simulink model "TP7"  (R2023b)
settings: Solver=VariableStepAuto  StartTime=0.0  StopTime=0.4  RelTol=1e-3
libraries: spsMosfetLib x6, spsSeriesRLCBranchLib x3, spsVoltageMeasurementLib x3, spsGroundLib x2, spsDCVoltageSourceLib x1, dspstat3 x1, sps_lib x1
settings Model: Creator=HP  LastModifiedBy=HP

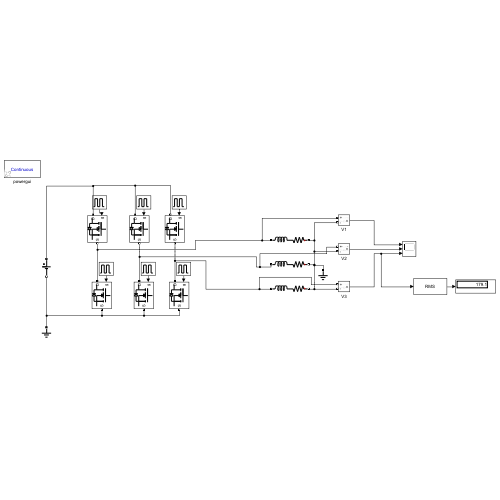
[thumbnail: Simulink's stored preview of the top-level diagram]
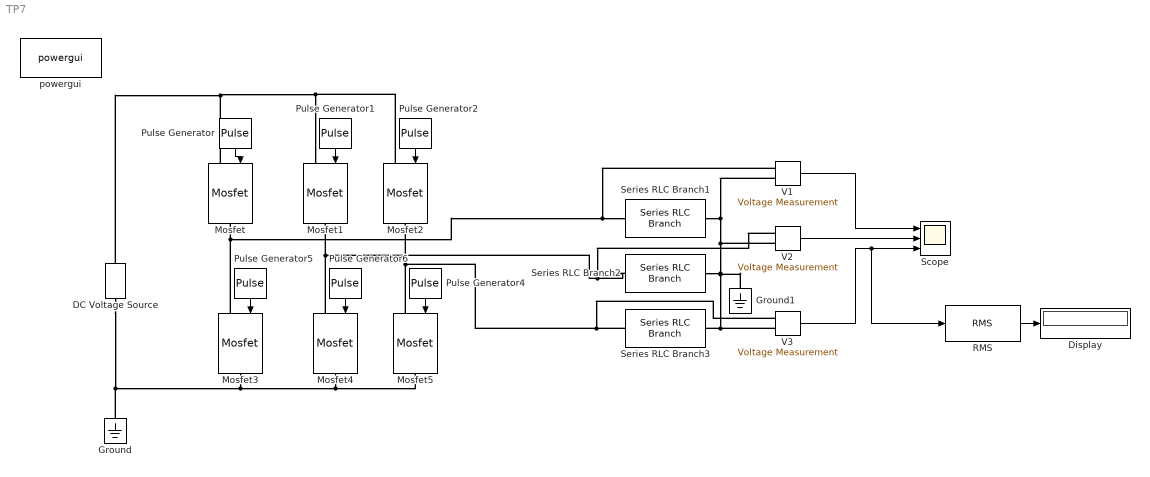
== system TP7 ==
  DC Voltage Source : spsDCVoltageSourceLib/DC Voltage Source  Amplitude=180  Measurements=None
  Display : Display
  Ground : spsGroundLib/Ground  LConnTagsString=a
  Ground1 : spsGroundLib/Ground  LConnTagsString=a
  Mosfet{,1..5} (6 alike) : spsMosfetLib/Mosfet  Ron=0.1  Lon=0  Rd=0.01  Vfd=0  IC=0  Rs=1e5  Cs=inf  Measurements=off
  Pulse Generator : DiscretePulseGenerator  PulseType=Time based  Period=0.002  PulseWidth=50  VectorParams1D=off
  Pulse Generator1 : DiscretePulseGenerator  PulseType=Time based  Period=0.002  PulseWidth=50  PhaseDelay=(.002*120)/360  VectorParams1D=off
  Pulse Generator2 : DiscretePulseGenerator  PulseType=Time based  Period=0.002  PulseWidth=50  PhaseDelay=(.002*240)/360  VectorParams1D=off
  Pulse Generator4 : DiscretePulseGenerator  PulseType=Time based  Period=0.002  PulseWidth=50  PhaseDelay=.002*(60/360)  VectorParams1D=off
  Pulse Generator5 : DiscretePulseGenerator  PulseType=Time based  Period=0.002  PulseWidth=50  PhaseDelay=(.002*180)/360  VectorParams1D=off
  Pulse Generator6 : DiscretePulseGenerator  PulseType=Time based  Period=0.002  PulseWidth=50  PhaseDelay=(.002*300)/360  VectorParams1D=off
  RMS : dspstat3/RMS  run=off  directionMode=Each column  dimension=1  InputProcessing=Columns as channels (frame based)  reset_popup=None
  Scope : Scope  NumInputPorts=3
  Series RLC Branch1 : spsSeriesRLCBranchLib/Series RLC Branch  LConnTagsString=__new0  RConnTagsString=__new0  BranchType=RL  Resistance=10  Inductance=40e-03  SetiL0=off  InitialCurrent=0  Capacitance=1e-6  Setx0=off  InitialVoltage=0  Measurements=None
  Series RLC Branch2 : spsSeriesRLCBranchLib/Series RLC Branch  LConnTagsString=__new0  RConnTagsString=__new0  BranchType=RL  Resistance=10  Inductance=40e-03  SetiL0=off  InitialCurrent=0  Capacitance=1e-6  Setx0=off  InitialVoltage=0  Measurements=None
  Series RLC Branch3 : spsSeriesRLCBranchLib/Series RLC Branch  LConnTagsString=__new0  RConnTagsString=__new0  BranchType=RL  Resistance=10  Inductance=40e-03  SetiL0=off  InitialCurrent=0  Capacitance=1e-6  Setx0=off  InitialVoltage=0  Measurements=None
  V1 : spsVoltageMeasurementLib/Voltage Measurement  PhasorSimulation=off  OutputType=Complex  PSBequivalent=0
  V2 : spsVoltageMeasurementLib/Voltage Measurement  PhasorSimulation=off  OutputType=Complex  PSBequivalent=0
  V3 : spsVoltageMeasurementLib/Voltage Measurement  PhasorSimulation=off  OutputType=Complex  PSBequivalent=0
  powergui : sps_lib/powergui  Priority=1  SimulationMode=Continuous  SampleTime=50e-6  frequency=60  Iterations=50  frequencyindice=0  Pbase=100e6  ErrMax=1e-4  UnitsV=kV  UnitsW=MW  buscounter=0  FunctionMessages=off  echomessages=off  EnableUseOfTLC=off  CurrentSourceSwitches=off  DisableSnubberDevices=off  DisableRonSwitches=off  DisableVfSwitches=off  DisplayEquations=off  AutomaticDiscreteSolvers=off  SolverType=Tustin/Backward Euler (TBE)  Interpol=off  ExternalGateDelay=off  methode=off  Ts=100  x0status=blocks  SPID=on  SwTol=0  HookPort=off  NonlinearTolerance=1e-4  nMaxIteration=100  ContinueOnMaxIteration=off  RestoreLinks=warning  ResistiveCurrentMeasurement=off  Frange=[0:2:500]  Ylog=off  Xlog=on  ShowGrid=off  save=off  variable=ZData  structure=0  ZoomFFT=off  StartTime=0.0  cycles=1  DisplayStyle=1  fundamental=60  FreqAxis=off  MaxFrequency=1000  frequencyindicesteady=1  RmsSteady=1  display=off
  wires:
  Pulse Generator/1 -> Mosfet/1
  Pulse Generator1/1 -> Mosfet1/1
  Pulse Generator2/1 -> Mosfet2/1
  Pulse Generator4/1 -> Mosfet5/1
  Pulse Generator5/1 -> Mosfet3/1
  Pulse Generator6/1 -> Mosfet4/1
  V1/1 -> Scope/1
  V2/1 -> Scope/2
  V3/1 -> RMS/1, Scope/3
  RMS/1 -> Display/1
  connections:
  Series RLC Branch1/LConn1 -- V3/LConn2 -- Series RLC Branch3/LConn1 -- Ground1/LConn1 -- Series RLC Branch2/LConn1 -- V2/LConn2 -- V1/LConn2
  Mosfet5/LConn1 -- V3/LConn1 -- Series RLC Branch3/RConn1 -- Mosfet2/RConn1
  Mosfet4/LConn1 -- V2/LConn1 -- Series RLC Branch2/RConn1 -- Mosfet1/RConn1
  Mosfet/RConn1 -- Mosfet3/LConn1 -- V1/LConn1 -- Series RLC Branch1/RConn1
  Mosfet/LConn1 -- DC Voltage Source/RConn1 -- Mosfet1/LConn1 -- Mosfet2/LConn1
  Mosfet3/RConn1 -- DC Voltage Source/LConn1 -- Ground/LConn1 -- Mosfet4/RConn1 -- Mosfet5/RConn1
